simulink model "ProjectSimulation"  (Simulink 7.6)
settings: Solver=ode23tb  StartTime=0.0  StopTime=1  RelTol=1e-3
libraries: powerlib x17, simulink x1
settings Model: Creator=rajpoppy  LastModifiedBy=Dinesh
settings DebuggingCC: FcnCallInpInsideContextMsg=Enable All
settings GRTTargetCC: CombineOutputUpdateFcns=on

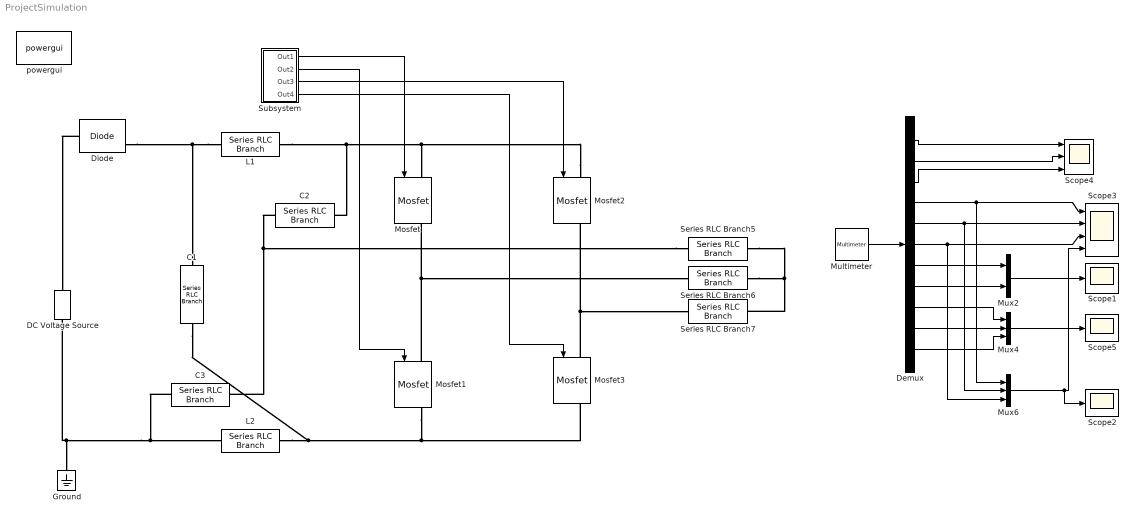
== system ProjectSimulation ==
  C1 : powerlib/Elements/Series RLC Branch  DialogController=POWERSYS.PowerSysDialog  PhysicalDomain=powersysdomain  SubClassName=unknown  LeftPortType=p1  RightPortType=p1  LConnTagsString=__new0  RConnTagsString=__new0  BranchType=C  Resistance=1  Inductance=1e-3  SetiL0=off  InitialCurrent=0  Capacitance=235e-6  Setx0=off  InitialVoltage=0  Measurements=Branch voltage
  C2 : powerlib/Elements/Series RLC Branch  DialogController=POWERSYS.PowerSysDialog  PhysicalDomain=powersysdomain  SubClassName=unknown  LeftPortType=p1  RightPortType=p1  LConnTagsString=__new0  RConnTagsString=__new0  BranchType=C  Resistance=1  Inductance=1e-3  SetiL0=off  InitialCurrent=0  Capacitance=470e-6  Setx0=off  InitialVoltage=0  Measurements=Branch voltage
  C3 : powerlib/Elements/Series RLC Branch  DialogController=POWERSYS.PowerSysDialog  PhysicalDomain=powersysdomain  SubClassName=unknown  LeftPortType=p1  RightPortType=p1  LConnTagsString=__new0  RConnTagsString=__new0  BranchType=C  Resistance=1  Inductance=1e-3  SetiL0=off  InitialCurrent=0  Capacitance=470e-6  Setx0=off  InitialVoltage=0  Measurements=Branch voltage
  DC Voltage Source : powerlib/Electrical Sources/DC Voltage Source  DialogController=POWERSYS.PowerSysDialog  SystemSampleTime=-1  Amplitude=90  Measurements=None
  Demux : Demux  Outputs=11
  Diode : powerlib/Power Electronics/Diode  DialogController=POWERSYS.PowerSysDialog  SystemSampleTime=-1  Ron=0.001  Lon=0  Vf=0.8  IC=0  UseSnubber=off  Rs=500  Cs=250e-9  Measurements=on
  Ground : powerlib/Elements/Ground  DialogController=POWERSYS.PowerSysDialog  PhysicalDomain=powersysdomain  SubClassName=unknown  LeftPortType=p1  RightPortType=p1  LConnTagsString=a
  L1 : powerlib/Elements/Series RLC Branch  DialogController=POWERSYS.PowerSysDialog  PhysicalDomain=powersysdomain  SubClassName=unknown  LeftPortType=p1  RightPortType=p1  LConnTagsString=__new0  RConnTagsString=__new0  BranchType=RL  Resistance=1  Inductance=6.4e-3  SetiL0=off  InitialCurrent=0  Capacitance=1e-6  Setx0=off  InitialVoltage=0  Measurements=Branch current
  L2 : powerlib/Elements/Series RLC Branch  DialogController=POWERSYS.PowerSysDialog  PhysicalDomain=powersysdomain  SubClassName=unknown  LeftPortType=p1  RightPortType=p1  LConnTagsString=__new0  RConnTagsString=__new0  BranchType=RL  Resistance=1  Inductance=6.4e-3  SetiL0=off  InitialCurrent=0  Capacitance=1e-6  Setx0=off  InitialVoltage=0  Measurements=Branch current
  Mosfet{,1..3} (4 alike) : powerlib/Power Electronics/Mosfet  DialogController=POWERSYS.PowerSysDialog  SystemSampleTime=-1  Ron=0.1  Lon=0  Rd=0.01  Vfd=0  IC=0  Rs=1e5  Cs=inf  Measurements=on
  Multimeter : powerlib/Measurements/Multimeter  SystemSampleTime=-1  PhasorSimulation=off  OutputType=Complex  sel=[4 5 6 9 10 11 7 8 1 2 3]  L=11  Gain=[1 1 1 1 1 1 1 1 1 1 1]  yselected={'Ub: Series RLC Branch5','Ub: Series RLC Branch6','Ub: Series RLC Branch7','Ib: Series RLC Branch5','Ib: Series RLC Branch6','Ib: Series RLC Branch7','Ib: L1','Ib: L2','Ub: C1','Ub: C2','Ub: C3'};  PSBOutputType=1  PSBequivalent=0  AxesSetting=[0,0.1,-100,100]  Display=0  SavedBlockNames=-11
  Mux2 : Mux  Inputs=2
  Mux4 : Mux  Inputs=3
  Mux6 : Mux  Inputs=3
  Scope1 : Scope
      settings: YMin=-4  SaveName=ScopeData4
  Scope2 : Scope
      settings: YMin=-20  YMax=200  SaveName=ScopeData5
  Scope3 : Scope  NumInputPorts=4
      settings: YMin=-3.5~-7~-7~-5  YMax=4.5~8~8~5  SaveName=ScopeData6
  Scope4 : Scope  NumInputPorts=3
      settings: YMin=-4~-1~-5  YMax=5~1~5
  Scope5 : Scope
      settings: YMin=-20  YMax=200  SaveName=ScopeData7
  Series RLC Branch5 : powerlib/Elements/Series RLC Branch  DialogController=POWERSYS.PowerSysDialog  PhysicalDomain=powersysdomain  SubClassName=unknown  LeftPortType=p1  RightPortType=p1  LConnTagsString=__new0  RConnTagsString=__new0  BranchType=RL  Resistance=10.5  Inductance=20.1e-3  SetiL0=off  InitialCurrent=0  Capacitance=1e-6  Setx0=off  InitialVoltage=0  Measurements=Branch voltage and current
  Series RLC Branch6 : powerlib/Elements/Series RLC Branch  DialogController=POWERSYS.PowerSysDialog  PhysicalDomain=powersysdomain  SubClassName=unknown  LeftPortType=p1  RightPortType=p1  LConnTagsString=__new0  RConnTagsString=__new0  BranchType=RL  Resistance=10.6  Inductance=18.4e-3  SetiL0=off  InitialCurrent=0  Capacitance=1e-6  Setx0=off  InitialVoltage=0  Measurements=Branch voltage and current
  Series RLC Branch7 : powerlib/Elements/Series RLC Branch  DialogController=POWERSYS.PowerSysDialog  PhysicalDomain=powersysdomain  SubClassName=unknown  LeftPortType=p1  RightPortType=p1  LConnTagsString=__new0  RConnTagsString=__new0  BranchType=RL  Resistance=10.2  Inductance=17.7e-3  SetiL0=off  InitialCurrent=0  Capacitance=1e-6  Setx0=off  InitialVoltage=0  Measurements=Branch voltage and current
  Subsystem : Subsystem
  powergui : powerlib/powergui  Priority=1  SystemSampleTime=-1  SimulationMode=Discrete  SampleTime=5e-6  frequency=60  SPID=off  DisableSnubberDevices=off  DisableRonSwitches=off  DisableVfSwitches=off  SwTol=0  Interpol=off  frequencyindice=0  echomessages=off  HookPort=off  DisplayEquations=off  FunctionMessages=off  EnableUseOfTLC=off  x0status=blocks  RestoreLinks=warning  ResistiveCurrentMeasurement=off  Ylog=off  Xlog=on  ShowGrid=off  save=off  variable=ZData  structure=ScopeData6  ZoomFFT=off  StartTime=0.8  cycles=3  DisplayStyle=1  fundamental=50  FreqAxis=off  MaxFrequency=1000  frequencyindicesteady=1  display=off  methode=off
  wires:
  Multimeter/1 -> Demux/1
  Demux/10 -> Mux4/2
  Demux/9 -> Mux4/1
  Demux/8 -> Mux2/2
  Demux/7 -> Mux2/1
  Mux2/1 -> Scope1/1
  Mux4/1 -> Scope5/1
  Demux/11 -> Mux4/3
  Subsystem/3(Out3) -> Mosfet2/1
  Subsystem/4(Out4) -> Mosfet3/1
  Demux/1 -> Scope4/1
  Demux/2 -> Scope4/2
  Demux/3 -> Scope4/3
  Demux/4 -> Scope3/1, Mux6/1
  Demux/5 -> Scope3/2, Mux6/2
  Demux/6 -> Scope3/3, Mux6/3
  Subsystem/2(Out2) -> Mosfet1/1
  Subsystem/1(Out1) -> Mosfet/1
  Mux6/1 -> Scope3/4, Scope2/1
  connections:
  Mosfet3/RConn1 -- Mosfet1/RConn1 -- C1/RConn1 -- L2/LConn1
  C3/RConn1 -- L2/RConn1 -- DC Voltage Source/LConn1 -- Ground/LConn1
  Mosfet1/LConn1 -- Mosfet/RConn1 -- Series RLC Branch6/LConn1
  Mosfet3/LConn1 -- Mosfet2/RConn1 -- Series RLC Branch7/LConn1
  Series RLC Branch6/RConn1 -- Series RLC Branch7/RConn1 -- Series RLC Branch5/RConn1
  L1/LConn1 -- C1/LConn1 -- Diode/RConn1
  Mosfet2/LConn1 -- Mosfet/LConn1 -- L1/RConn1 -- C2/LConn1
  Series RLC Branch5/LConn1 -- C2/RConn1 -- C3/LConn1
  Diode/LConn1 -- DC Voltage Source/RConn1

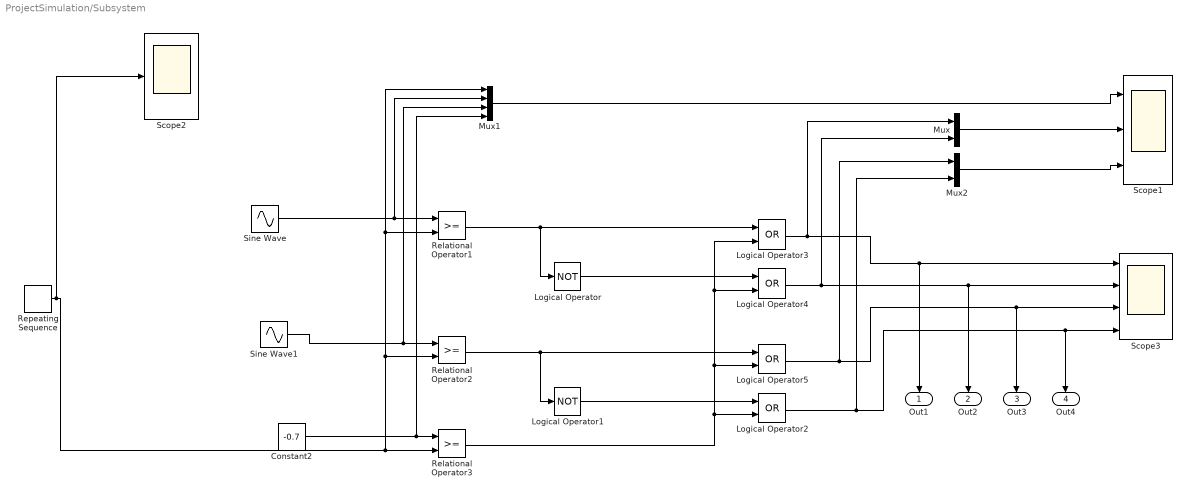
== system ProjectSimulation/Subsystem ==
  Constant2 : Constant  Value=-0.7
  Logical Operator : Logic  Operator=NOT  AllPortsSameDT=off  OutDataTypeStr=boolean
  Logical Operator1 : Logic  Operator=NOT  AllPortsSameDT=off  OutDataTypeStr=boolean
  Logical Operator{2..5} (4 alike) : Logic  Operator=OR  AllPortsSameDT=off  OutDataTypeStr=boolean
  Mux : Mux  Inputs=2
  Mux1 : Mux
  Mux2 : Mux  Inputs=2
  Relational Operator1 : RelationalOperator  OutDataTypeStr=boolean
  Relational Operator2 : RelationalOperator  OutDataTypeStr=boolean
  Relational Operator3 : RelationalOperator  OutDataTypeStr=boolean
  Repeating Sequence : simulink/Sources/Repeating Sequence  SystemSampleTime=-1  rep_seq_t=[0 0.5 1 1.5 2]*(1/(10000))  rep_seq_y=[-1 1 -1 1 -1]
  Scope1 : Scope  NumInputPorts=3
      settings: YMin=-4~-1~-5  YMax=5~5~5
  Scope2 : Scope
      settings: YMin=0  SaveName=ScopeData2
  Scope3 : Scope  NumInputPorts=4
      settings: YMin=0~0~-5~0  YMax=5~5~5~5  SaveName=ScopeData3
  Sine Wave : Sin  Amplitude=0.8  Frequency=2*pi*50  Phase=2*pi/3  SampleTime=0
  Sine Wave1 : Sin  Amplitude=0.7  Frequency=2*pi*50  Phase=4*pi/3  SampleTime=0
  Out1 : Outport
  Out2 : Outport  Port=2
  Out3 : Outport  Port=3
  Out4 : Outport  Port=4
  wires:
  Relational Operator1/1 -> Logical Operator/1, Logical Operator3/1
  Relational Operator2/1 -> Logical Operator1/1, Logical Operator5/1
  Repeating Sequence/1 -> Scope2/1, Relational Operator3/2, Relational Operator2/2, Relational Operator1/2, Mux1/1
  Constant2/1 -> Relational Operator3/1, Mux1/4
  Sine Wave1/1 -> Relational Operator2/1, Mux1/3
  Sine Wave/1 -> Relational Operator1/1, Mux1/2
  Logical Operator/1 -> Logical Operator4/1
  Logical Operator1/1 -> Logical Operator2/1
  Relational Operator3/1 -> Logical Operator3/2, Logical Operator4/2, Logical Operator5/2, Logical Operator2/2
  Logical Operator3/1 -> Mux/1, Scope3/1, Out1/1
  Logical Operator4/1 -> Mux/2, Scope3/2, Out2/1
  Logical Operator5/1 -> Mux2/1, Scope3/3, Out3/1
  Logical Operator2/1 -> Mux2/2, Scope3/4, Out4/1
  Mux1/1 -> Scope1/1
  Mux/1 -> Scope1/2
  Mux2/1 -> Scope1/3
